simulink model "hdlcoder_dwt"  (R2021b)
settings: Solver=FixedStepDiscrete  StartTime=0.0  StopTime=15000  RelTol=1e-3
model workspace (MAT data in the model file):
  out_size = 0
settings Model: DataTypeOverride=Off  SimulationMode=accelerator  Creator=local_adm  LastModifiedBy=local_adm
settings SolverCC: AlgebraicLoopSolver=TrustRegion  AutoInsertRateTranBlk=on
settings DataIOCC: LimitDataPoints=on  SaveOutput=off  SaveTime=off
settings OptimizationCC: BlockReduction=off  ConditionallyExecuteInputs=off  DefaultParameterBehavior=Inlined  LifeSpan=inf
settings DebuggingCC: AlgebraicLoopMsg=error  SingleTaskRateTransMsg=error  ParameterPrecisionLossMsg=none  AllowSymbolicDim=off  StrictBusMsg=ErrorOnBusTreatedAsVector  SFUnexpectedBacktrackingDiag=warning  SFNoUnconditionalDefaultTransitionDiag=warning  SFExecutionAtInitializationDiag=none  SFMachineParentedDataDiag=warning  ArithmeticOperatorsInVariantConditions=warning
settings HardwareCC: ProdBitPerPointer=32  ProdBitPerSizeT=32  ProdBitPerPtrDiffT=32  ProdLargestAtomicFloat=None  ProdIntDivRoundTo=Undefined  ProdEndianess=Unspecified  ProdWordSize=32  ProdHWDeviceType=ASIC/FPGA->ASIC/FPGA  ProdEqTarget=off
settings SFSimCC: SimUseLocalCustomCode=off  CustomCodeUndefinedFunction=UseInterfaceOnly
settings RTWCC: RTWUseLocalCustomCode=off
settings CodeAppCC: StateflowObjectComments=on
settings GRTTargetCC: TargetLangStandard=C89/C90 (ANSI)
settings ConfigComp: CovScope=ReferencedModels  CovMetricSettings=dw  CovSaveCumulativeToWorkspaceVar=on  CovSaveSingleToWorkspaceVar=on  CovExternalEMLEnable=off  CovSFcnEnable=off

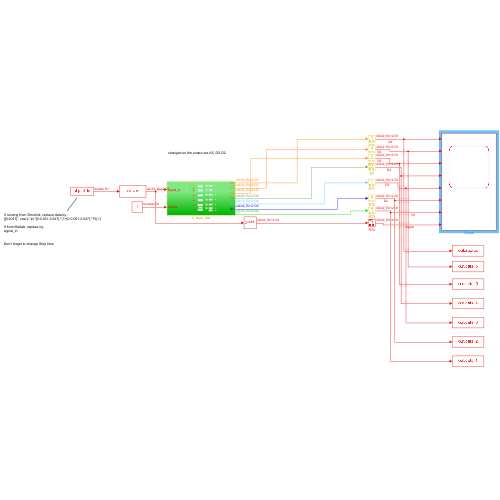
[thumbnail: Simulink's stored preview of the top-level diagram]
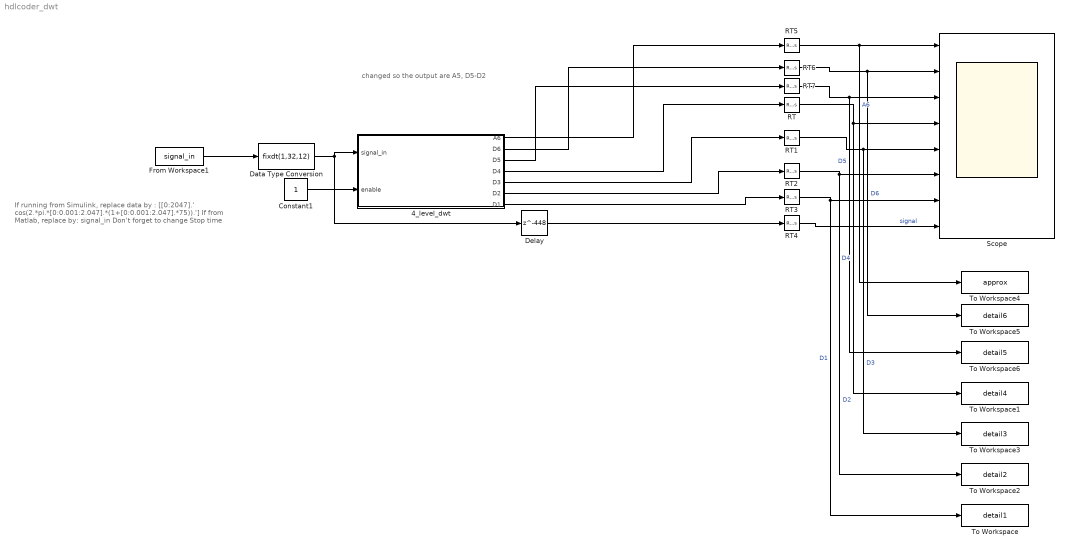
== system hdlcoder_dwt ==
  note: changed so the output are A5, D5-D2
  note: If running from Simulink, replace data by :
      | [[0:2047].' cos(2.*pi.*[0:0.001:2.047].*(1+[0:0.001:2.047].*75)).']
      |
      | If from Matlab, replace by:
      | signal_in
      |
      |
      | Don't forget to change Stop time
  4_level_dwt : Subsystem
  Constant1 : Constant  OutDataTypeStr=boolean  SampleTime=1
  Data Type Conversion : DataTypeConversion  OutMax=2  OutDataTypeStr=fixdt(1,32,12)
  Delay : Delay  DelayLength=448
  From Workspace1 : FromWorkspace  VariableName=signal_in  SampleTime=1  OutputAfterFinalValue=Setting to zero
  RT{,1..7} (8 alike) : RateTransition  OutPortSampleTime=1
  Scope : Scope  NumInputPorts=8
  To Workspace : ToWorkspace  VariableName=detail1  SampleTime=-1
  To Workspace1 : ToWorkspace  VariableName=detail4  SampleTime=-1
  To Workspace2 : ToWorkspace  VariableName=detail2  SampleTime=-1
  To Workspace3 : ToWorkspace  VariableName=detail3  SampleTime=-1
  To Workspace4 : ToWorkspace  VariableName=approx  SampleTime=-1
  To Workspace5 : ToWorkspace  VariableName=detail6  SampleTime=-1
  To Workspace6 : ToWorkspace  VariableName=detail5  SampleTime=-1
  wires:
  Constant1/1 -> 4_level_dwt/2(enable)
  Data Type Conversion/1 -> Delay/1, 4_level_dwt/1(signal_in)
  RT/1 -> Scope/4, To Workspace1/1  "D4"
  RT1/1 -> To Workspace3/1, Scope/5  "D3"
  RT2/1 -> To Workspace2/1, Scope/6  "D2"
  RT3/1 -> To Workspace/1, Scope/7  "D1"
  RT4/1 -> Scope/8  "signal"
  RT5/1 -> To Workspace4/1, Scope/1  "A6"
  4_level_dwt/7(D1) -> RT3/1
  4_level_dwt/6(D2) -> RT2/1
  4_level_dwt/5(D3) -> RT1/1
  4_level_dwt/4(D4) -> RT/1
  4_level_dwt/1(A6) -> RT5/1
  From Workspace1/1 -> Data Type Conversion/1
  RT6/1 -> To Workspace5/1, Scope/2  "D6"
  RT7/1 -> To Workspace6/1, Scope/3  "D5"
  4_level_dwt/2(D6) -> RT6/1
  4_level_dwt/3(D5) -> RT7/1
  Delay/1 -> RT4/1

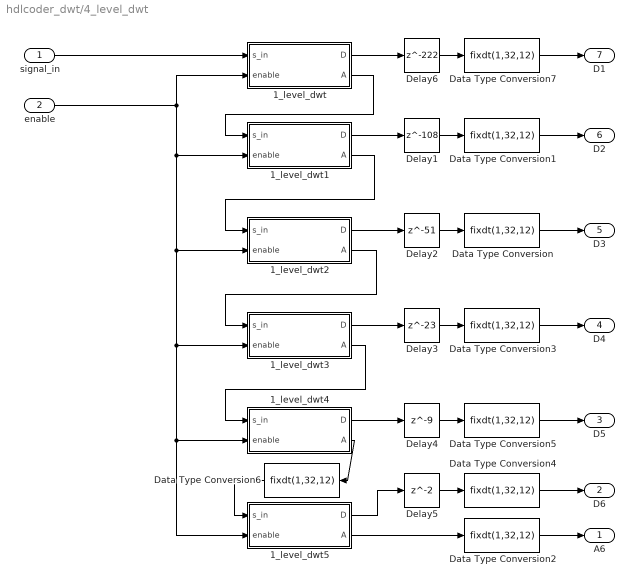
== system hdlcoder_dwt/4_level_dwt ==
  signal_in : Inport
  enable : Inport  Port=2
  1_level_dwt : Subsystem
  1_level_dwt1 : Subsystem
  1_level_dwt2 : Subsystem
  1_level_dwt3 : Subsystem
  1_level_dwt4 : Subsystem
  1_level_dwt5 : Subsystem
  Data Type Conversion{,1..7} (8 alike) : DataTypeConversion  OutDataTypeStr=fixdt(1,32,12)
  Delay1 : Delay  DelayLength=108
  Delay2 : Delay  DelayLength=51
  Delay3 : Delay  DelayLength=23
  Delay4 : Delay  DelayLength=9
  Delay5 : Delay
  Delay6 : Delay  DelayLength=222
  A6 : Outport  VectorParamsAs1DForOutWhenUnconnected=off
  D6 : Outport  Port=2  VectorParamsAs1DForOutWhenUnconnected=off
  D5 : Outport  Port=3  VectorParamsAs1DForOutWhenUnconnected=off
  D4 : Outport  Port=4  VectorParamsAs1DForOutWhenUnconnected=off
  D3 : Outport  Port=5  VectorParamsAs1DForOutWhenUnconnected=off
  D2 : Outport  Port=6  VectorParamsAs1DForOutWhenUnconnected=off
  D1 : Outport  Port=7  VectorParamsAs1DForOutWhenUnconnected=off
  wires:
  signal_in/1 -> 1_level_dwt/1(s_in)
  enable/1 -> 1_level_dwt1/2(enable), 1_level_dwt5/2(enable), 1_level_dwt4/2(enable), 1_level_dwt3/2(enable), 1_level_dwt2/2(enable), 1_level_dwt/2(enable)
  1_level_dwt/2(A) -> 1_level_dwt1/1(s_in)
  1_level_dwt1/2(A) -> 1_level_dwt2/1(s_in)
  1_level_dwt2/2(A) -> 1_level_dwt3/1(s_in)
  1_level_dwt1/1(D) -> Delay1/1
  1_level_dwt2/1(D) -> Delay2/1
  1_level_dwt3/1(D) -> Delay3/1
  Delay2/1 -> Data Type Conversion/1
  Delay1/1 -> Data Type Conversion1/1
  Delay3/1 -> Data Type Conversion3/1
  1_level_dwt3/2(A) -> 1_level_dwt4/1(s_in)
  Delay4/1 -> Data Type Conversion5/1
  1_level_dwt4/1(D) -> Delay4/1
  1_level_dwt5/1(D) -> Delay5/1
  1_level_dwt5/2(A) -> Data Type Conversion2/1
  Delay5/1 -> Data Type Conversion4/1
  Data Type Conversion2/1 -> A6/1
  Data Type Conversion1/1 -> D2/1
  Data Type Conversion/1 -> D3/1
  Data Type Conversion3/1 -> D4/1
  Data Type Conversion4/1 -> D6/1
  Data Type Conversion5/1 -> D5/1
  1_level_dwt4/2(A) -> Data Type Conversion6/1
  Data Type Conversion6/1 -> 1_level_dwt5/1(s_in)
  Delay6/1 -> Data Type Conversion7/1
  1_level_dwt/1(D) -> Delay6/1
  Data Type Conversion7/1 -> D1/1

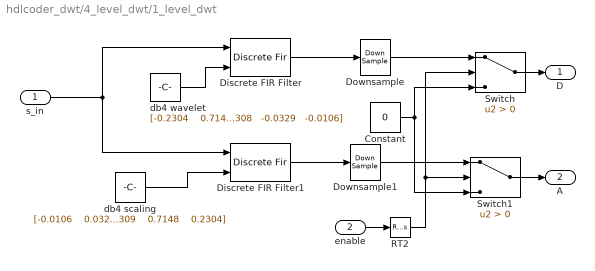
== system hdlcoder_dwt/4_level_dwt/1_level_dwt ==
  s_in : Inport
  enable : Inport  Port=2
  Constant : Constant  Value=0  OutDataTypeStr=Inherit: Inherit via back propagation
  Discrete FIR Filter : DiscreteFir  CoefSource=Input port
      settings: InputPortMap=u0,u1
  Discrete FIR Filter1 : DiscreteFir  CoefSource=Input port
      settings: InputPortMap=u0,u1
  Downsample : DownSample  phase=1  RateOptions=Allow multirate processing
  Downsample1 : DownSample  phase=1  RateOptions=Allow multirate processing
  RT2 : RateTransition  OutPortSampleTime=2
  Switch : Switch  Criteria=u2 > Threshold
  Switch1 : Switch  Criteria=u2 > Threshold
  db4 scaling : Constant  Value="[-0.0106    0.0329    0.0308   -0.1870   -0.0280    0.6309    0.7148    0.2304]"  OutDataTypeStr=Inherit: Inherit via back propagation
  db4 wavelet : Constant  Value="[-0.2304    0.7148   -0.6309   -0.0280    0.1870    0.0308   -0.0329   -0.0106]"  OutDataTypeStr=Inherit: Inherit via back propagation
  D : Outport
  A : Outport  Port=2
  wires:
  db4 wavelet/1 -> Discrete FIR Filter/2
  s_in/1 -> Discrete FIR Filter1/1, Discrete FIR Filter/1
  db4 scaling/1 -> Discrete FIR Filter1/2
  Constant/1 -> Switch/3, Switch1/3
  Discrete FIR Filter/1 -> Downsample/1
  Discrete FIR Filter1/1 -> Downsample1/1
  Switch1/1 -> A/1
  Switch/1 -> D/1
  Downsample/1 -> Switch/1
  Downsample1/1 -> Switch1/1
  enable/1 -> RT2/1
  RT2/1 -> Switch/2, Switch1/2

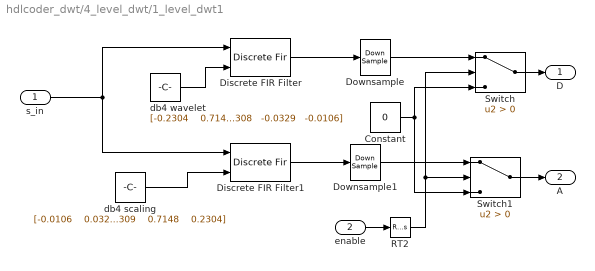
== system hdlcoder_dwt/4_level_dwt/1_level_dwt1 ==
  s_in : Inport
  enable : Inport  Port=2
  Constant : Constant  Value=0  OutDataTypeStr=Inherit: Inherit via back propagation
  Discrete FIR Filter : DiscreteFir  CoefSource=Input port
      settings: InputPortMap=u0,u1
  Discrete FIR Filter1 : DiscreteFir  CoefSource=Input port
      settings: InputPortMap=u0,u1
  Downsample : DownSample  phase=1  RateOptions=Allow multirate processing
  Downsample1 : DownSample  phase=1  RateOptions=Allow multirate processing
  RT2 : RateTransition  OutPortSampleTime=4
  Switch : Switch  Criteria=u2 > Threshold
  Switch1 : Switch  Criteria=u2 > Threshold
  db4 scaling : Constant  Value="[-0.0106    0.0329    0.0308   -0.1870   -0.0280    0.6309    0.7148    0.2304]"  OutDataTypeStr=Inherit: Inherit via back propagation
  db4 wavelet : Constant  Value="[-0.2304    0.7148   -0.6309   -0.0280    0.1870    0.0308   -0.0329   -0.0106]"  OutDataTypeStr=Inherit: Inherit via back propagation
  D : Outport
  A : Outport  Port=2
  wires:
  db4 wavelet/1 -> Discrete FIR Filter/2
  s_in/1 -> Discrete FIR Filter1/1, Discrete FIR Filter/1
  db4 scaling/1 -> Discrete FIR Filter1/2
  Constant/1 -> Switch/3, Switch1/3
  Discrete FIR Filter/1 -> Downsample/1
  Discrete FIR Filter1/1 -> Downsample1/1
  Switch1/1 -> A/1
  Switch/1 -> D/1
  Downsample/1 -> Switch/1
  Downsample1/1 -> Switch1/1
  enable/1 -> RT2/1
  RT2/1 -> Switch/2, Switch1/2

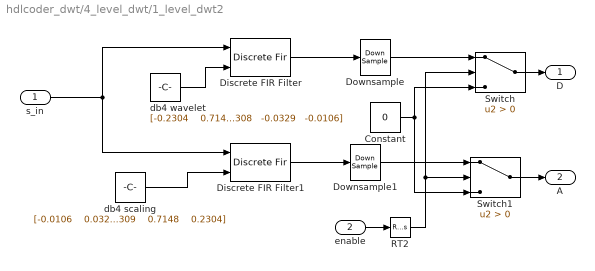
== system hdlcoder_dwt/4_level_dwt/1_level_dwt2 ==
  s_in : Inport
  enable : Inport  Port=2
  Constant : Constant  Value=0  OutDataTypeStr=Inherit: Inherit via back propagation
  Discrete FIR Filter : DiscreteFir  CoefSource=Input port
      settings: InputPortMap=u0,u1
  Discrete FIR Filter1 : DiscreteFir  CoefSource=Input port
      settings: InputPortMap=u0,u1
  Downsample : DownSample  phase=1  RateOptions=Allow multirate processing
  Downsample1 : DownSample  phase=1  RateOptions=Allow multirate processing
  RT2 : RateTransition  OutPortSampleTime=8
  Switch : Switch  Criteria=u2 > Threshold
  Switch1 : Switch  Criteria=u2 > Threshold
  db4 scaling : Constant  Value="[-0.0106    0.0329    0.0308   -0.1870   -0.0280    0.6309    0.7148    0.2304]"  OutDataTypeStr=Inherit: Inherit via back propagation
  db4 wavelet : Constant  Value="[-0.2304    0.7148   -0.6309   -0.0280    0.1870    0.0308   -0.0329   -0.0106]"  OutDataTypeStr=Inherit: Inherit via back propagation
  D : Outport
  A : Outport  Port=2
  wires:
  db4 wavelet/1 -> Discrete FIR Filter/2
  s_in/1 -> Discrete FIR Filter1/1, Discrete FIR Filter/1
  db4 scaling/1 -> Discrete FIR Filter1/2
  Constant/1 -> Switch/3, Switch1/3
  Discrete FIR Filter/1 -> Downsample/1
  Discrete FIR Filter1/1 -> Downsample1/1
  Switch1/1 -> A/1
  Switch/1 -> D/1
  Downsample/1 -> Switch/1
  Downsample1/1 -> Switch1/1
  enable/1 -> RT2/1
  RT2/1 -> Switch/2, Switch1/2

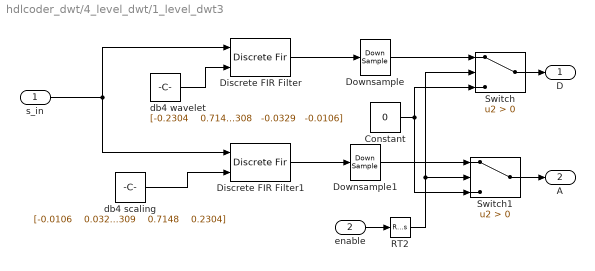
== system hdlcoder_dwt/4_level_dwt/1_level_dwt3 ==
  s_in : Inport
  enable : Inport  Port=2
  Constant : Constant  Value=0  OutDataTypeStr=Inherit: Inherit via back propagation
  Discrete FIR Filter : DiscreteFir  CoefSource=Input port
      settings: InputPortMap=u0,u1
  Discrete FIR Filter1 : DiscreteFir  CoefSource=Input port
      settings: InputPortMap=u0,u1
  Downsample : DownSample  phase=1  RateOptions=Allow multirate processing
  Downsample1 : DownSample  phase=1  RateOptions=Allow multirate processing
  RT2 : RateTransition  OutPortSampleTime=16
  Switch : Switch  Criteria=u2 > Threshold
  Switch1 : Switch  Criteria=u2 > Threshold
  db4 scaling : Constant  Value="[-0.0106    0.0329    0.0308   -0.1870   -0.0280    0.6309    0.7148    0.2304]"  OutDataTypeStr=Inherit: Inherit via back propagation
  db4 wavelet : Constant  Value="[-0.2304    0.7148   -0.6309   -0.0280    0.1870    0.0308   -0.0329   -0.0106]"  OutDataTypeStr=Inherit: Inherit via back propagation
  D : Outport
  A : Outport  Port=2
  wires:
  db4 wavelet/1 -> Discrete FIR Filter/2
  s_in/1 -> Discrete FIR Filter1/1, Discrete FIR Filter/1
  db4 scaling/1 -> Discrete FIR Filter1/2
  Constant/1 -> Switch/3, Switch1/3
  Discrete FIR Filter/1 -> Downsample/1
  Switch1/1 -> A/1
  Switch/1 -> D/1
  Downsample/1 -> Switch/1
  Downsample1/1 -> Switch1/1
  enable/1 -> RT2/1
  RT2/1 -> Switch/2, Switch1/2
  Discrete FIR Filter1/1 -> Downsample1/1

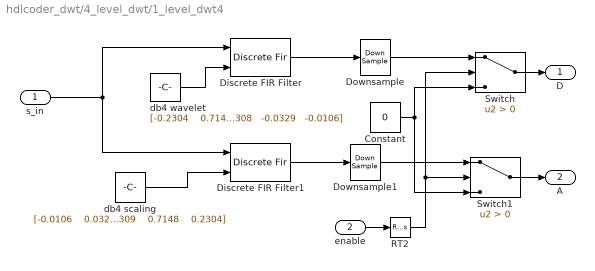
== system hdlcoder_dwt/4_level_dwt/1_level_dwt4 ==
  s_in : Inport
  enable : Inport  Port=2
  Constant : Constant  Value=0  OutDataTypeStr=Inherit: Inherit via back propagation
  Discrete FIR Filter : DiscreteFir  CoefSource=Input port
      settings: InputPortMap=u0,u1
  Discrete FIR Filter1 : DiscreteFir  CoefSource=Input port
      settings: InputPortMap=u0,u1
  Downsample : DownSample  phase=1  RateOptions=Allow multirate processing
  Downsample1 : DownSample  phase=1  RateOptions=Allow multirate processing
  RT2 : RateTransition  OutPortSampleTime=32
  Switch : Switch  Criteria=u2 > Threshold
  Switch1 : Switch  Criteria=u2 > Threshold
  db4 scaling : Constant  Value="[-0.0106    0.0329    0.0308   -0.1870   -0.0280    0.6309    0.7148    0.2304]"  OutDataTypeStr=Inherit: Inherit via back propagation
  db4 wavelet : Constant  Value="[-0.2304    0.7148   -0.6309   -0.0280    0.1870    0.0308   -0.0329   -0.0106]"  OutDataTypeStr=Inherit: Inherit via back propagation
  D : Outport
  A : Outport  Port=2
  wires:
  db4 wavelet/1 -> Discrete FIR Filter/2
  s_in/1 -> Discrete FIR Filter1/1, Discrete FIR Filter/1
  db4 scaling/1 -> Discrete FIR Filter1/2
  Constant/1 -> Switch/3, Switch1/3
  Discrete FIR Filter/1 -> Downsample/1
  Switch1/1 -> A/1
  Switch/1 -> D/1
  Downsample/1 -> Switch/1
  Downsample1/1 -> Switch1/1
  enable/1 -> RT2/1
  RT2/1 -> Switch/2, Switch1/2
  Discrete FIR Filter1/1 -> Downsample1/1

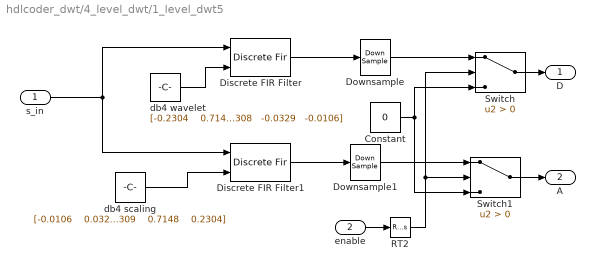
== system hdlcoder_dwt/4_level_dwt/1_level_dwt5 ==
  s_in : Inport
  enable : Inport  Port=2
  Constant : Constant  Value=0  OutDataTypeStr=Inherit: Inherit via back propagation
  Discrete FIR Filter : DiscreteFir  CoefSource=Input port
      settings: InputPortMap=u0,u1
  Discrete FIR Filter1 : DiscreteFir  CoefSource=Input port
      settings: InputPortMap=u0,u1
  Downsample : DownSample  phase=1  RateOptions=Allow multirate processing
  Downsample1 : DownSample  phase=1  RateOptions=Allow multirate processing
  RT2 : RateTransition  OutPortSampleTime=64
  Switch : Switch  Criteria=u2 > Threshold
  Switch1 : Switch  Criteria=u2 > Threshold
  db4 scaling : Constant  Value="[-0.0106    0.0329    0.0308   -0.1870   -0.0280    0.6309    0.7148    0.2304]"  OutDataTypeStr=Inherit: Inherit via back propagation
  db4 wavelet : Constant  Value="[-0.2304    0.7148   -0.6309   -0.0280    0.1870    0.0308   -0.0329   -0.0106]"  OutDataTypeStr=Inherit: Inherit via back propagation
  D : Outport
  A : Outport  Port=2
  wires:
  db4 wavelet/1 -> Discrete FIR Filter/2
  s_in/1 -> Discrete FIR Filter1/1, Discrete FIR Filter/1
  db4 scaling/1 -> Discrete FIR Filter1/2
  Constant/1 -> Switch/3, Switch1/3
  Discrete FIR Filter/1 -> Downsample/1
  Switch1/1 -> A/1
  Switch/1 -> D/1
  Downsample/1 -> Switch/1
  Downsample1/1 -> Switch1/1
  enable/1 -> RT2/1
  RT2/1 -> Switch/2, Switch1/2
  Discrete FIR Filter1/1 -> Downsample1/1
